simulink model "lab2"  (R2024b)
settings: Solver=VariableStepAuto  StartTime=0.0  StopTime=200  RelTol=1e-3
values from neighbouring files (symbols this model uses):
  b = 0.00002    (= 2e-05)    [Lab2.m]    (also in Last.m = 0.5; lab2_2.m = 25; untitled.m)
  J = 4*10^-6    (= 4e-06)    [Lab2.m]    (also in Last.m = 2; untitled.m)
  k = 10    [lab2_2.m]    (also in untitled.m)
  Kb = 0.04    [Lab2.m]    (also in Last.m = 0.1; untitled.m)
  Kt = 0.04    [Lab2.m]    (also in Last.m = 10; untitled.m)
  L = 1.2*10^-3    (= 0.0012)    [Lab2.m]    (also in untitled.m = 0.01)
  M = 200    [lab2_2.m]    (also in untitled.m)
  R = 8    [Lab2.m]    (also in untitled.m = 47000)
settings Model: Creator=Faizy  LastModifiedBy=Faizy

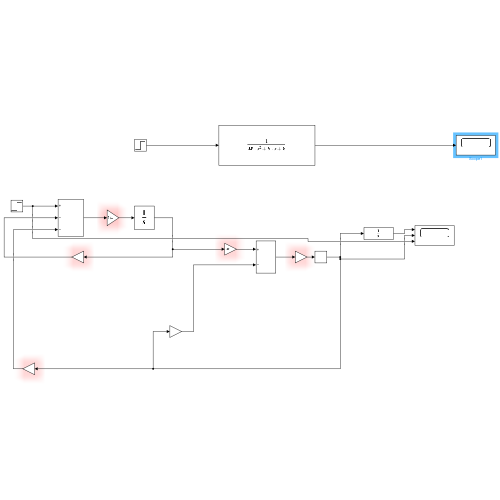
[thumbnail: Simulink's stored preview of the top-level diagram]
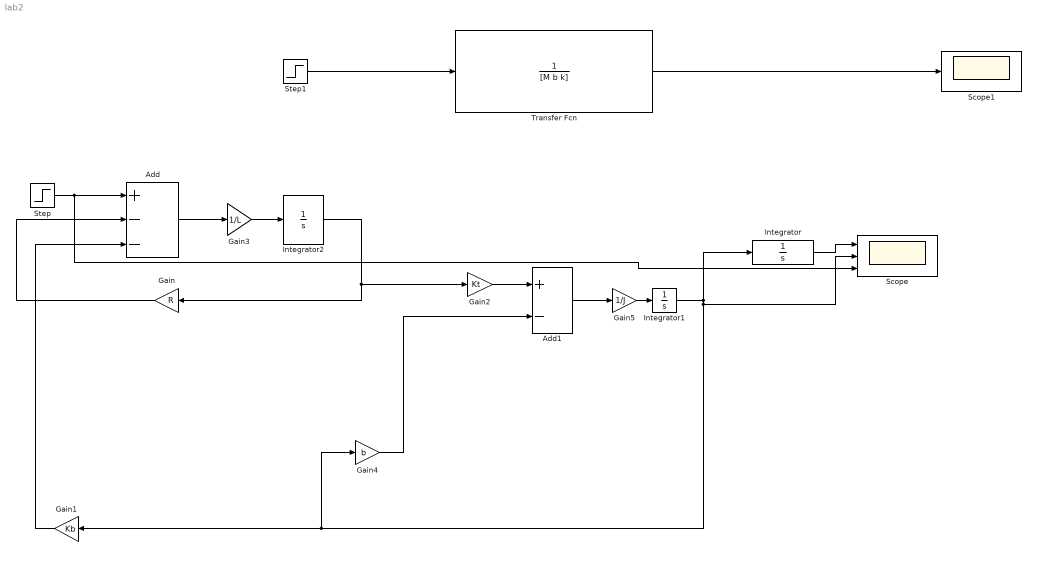
== system lab2 ==
  Add : Sum  Inputs=+--
  Add1 : Sum  Inputs=+-
  Gain : Gain  Gain=R
  Gain1 : Gain  Gain=Kb
  Gain2 : Gain  Gain=Kt
  Gain3 : Gain  Gain=1/L
  Gain4 : Gain  Gain=b
  Gain5 : Gain  Gain=1/J
  Integrator : Integrator
  Integrator1 : Integrator
  Integrator2 : Integrator
  Scope : Scope  NumInputPorts=3
  Scope1 : Scope
  Step : Step  SampleTime=0
  Step1 : Step  SampleTime=0
  Transfer Fcn : TransferFcn  Denominator=[M b k]
  wires:
  Transfer Fcn/1 -> Scope1/1
  Step1/1 -> Transfer Fcn/1
  Gain5/1 -> Integrator1/1
  Integrator2/1 -> Gain2/1, Gain/1
  Gain2/1 -> Add1/1
  Integrator1/1 -> Integrator/1, Scope/2, Gain4/1, Gain1/1
  Gain4/1 -> Add1/2
  Add/1 -> Gain3/1
  Gain1/1 -> Add/3
  Gain/1 -> Add/2
  Add1/1 -> Gain5/1
  Step/1 -> Scope/3, Add/1
  Integrator/1 -> Scope/1
  Gain3/1 -> Integrator2/1
